simulink model "DoubleTank_PID"  (Simulink 8.1)
settings: Solver=ode4  StartTime=0.0  StopTime=2000  FixedStep=0.5  RelTol=1e-3
PreLoadFcn:
  | pid6=readfis('pid6.fis')
InitFcn:
  | init
settings Model: Creator=Administrator  LastModifiedBy=Administrator
settings DataIOCC: SignalLoggingSaveFormat=Dataset
settings OptimizationCC: ExpressionDepthLimit=128
settings DebuggingCC: FcnCallInpInsideContextMsg=EnableAllAsError
settings GRTTargetCC: CombineOutputUpdateFcns=on  GRTInterface=off

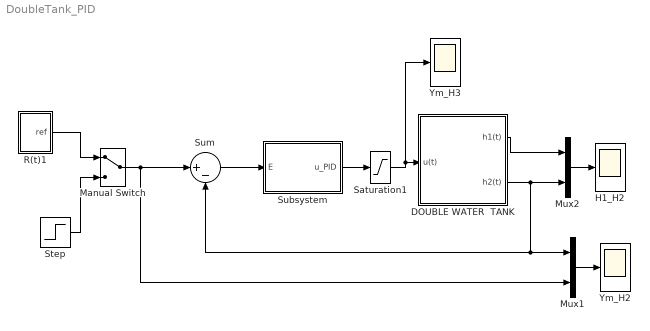
== system DoubleTank_PID ==
  DOUBLE WATER  TANK : Subsystem  mask(Input value){k=6, A_1=15.9043, A_2=15.9043, a1=0.3167, a2=0.1780, g=981}
      mask prompts: k "He so luu luong cua bom k"; A_1 "Tiet dien bon 1"; A_2 "Tiet dien bon 2"; a1 "tiet dien van xa 1"; a2 "tiet dien van xa 2"; g "Gia toc trong truong g"
      mask help: Please input behind values...
  H1_H2 : Scope
      settings: TimeRange=500  YMin=0  YMax=25  SaveName=h1
  Manual Switch : ManualSwitch
  Mux1 : Mux  Inputs=2
  Mux2 : Mux  Inputs=2
  R(t)1 : Subsystem
  Saturation1 : Saturate  UpperLimit=12  LowerLimit=0
  Step : Step  Time=0  After=25  SampleTime=0
  Subsystem : Subsystem  mask{Kp=5, Ki=0.5, Kd=0.1}
      mask prompts: Kp "He so Kp"; Ki "He so Ki"; Kd "He so Kd"
  Sum : Sum  Inputs=|+-
  Ym_H2 : Scope
      settings: TimeRange=500  YMin=38  YMax=42  SaveName=h
  Ym_H3 : Scope
      settings: TimeRange=500  YMin=0  YMax=25  SaveName=h2
  wires:
  Mux2/1 -> H1_H2/1
  R(t)1/1(ref) -> Manual Switch/1
  Step/1 -> Manual Switch/2
  Manual Switch/1 -> Sum/1, Mux1/2
  Subsystem/1(u_PID) -> Saturation1/1
  DOUBLE WATER  TANK/2(h2(t)) -> Mux2/2, Sum/2, Mux1/1
  DOUBLE WATER  TANK/1(h1(t)) -> Mux2/1
  Mux1/1 -> Ym_H2/1
  Saturation1/1 -> Ym_H3/1, DOUBLE WATER  TANK/1(u(t))
  Sum/1 -> Subsystem/1(E)

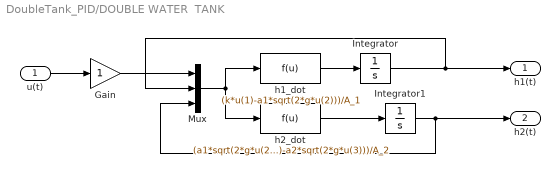
== system DoubleTank_PID/DOUBLE WATER  TANK ==
  u(t) : Inport
  Gain : Gain  SaturateOnIntegerOverflow=on  OutDataTypeStr=Inherit: Same as input  ParamDataTypeStr=Inherit: Same as input
  Integrator : Integrator  LimitOutput=on  UpperSaturationLimit=100  LowerSaturationLimit=0
  Integrator1 : Integrator  LimitOutput=on  UpperSaturationLimit=100  LowerSaturationLimit=0
  Mux : Mux  Inputs=3
  h1_dot : Fcn  Expr=(k*u(1)-a1*sqrt(2*g*u(2)))/A_1
  h2_dot : Fcn  Expr=(a1*sqrt(2*g*u(2))-a2*sqrt(2*g*u(3)))/A_2
  h1(t) : Outport
  h2(t) : Outport  Port=2
  wires:
  h2_dot/1 -> Integrator1/1
  Integrator/1 -> Mux/2, h1(t)/1
  h1_dot/1 -> Integrator/1
  Mux/1 -> h2_dot/1, h1_dot/1
  Integrator1/1 -> Mux/3, h2(t)/1
  u(t)/1 -> Gain/1
  Gain/1 -> Mux/1

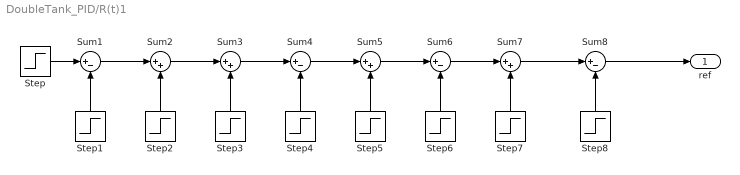
== system DoubleTank_PID/R(t)1 ==
  Step : Step  Time=0  After=15  SampleTime=0
  Step1 : Step  Time=250  After=5  SampleTime=0
  Step2 : Step  Time=500  After=5  SampleTime=0
  Step3 : Step  Time=750  After=15  SampleTime=0
  Step4 : Step  Time=1000  After=10  SampleTime=0
  Step5 : Step  Time=1250  After=15  SampleTime=0
  Step6 : Step  Time=1500  After=5  SampleTime=0
  Step7 : Step  Time=1750  After=15  SampleTime=0
  Step8 : Step  Time=2000  After=5  SampleTime=0
  Sum{1,4,6,8} (4 alike) : Sum  Inputs=|+-  SaturateOnIntegerOverflow=on
  Sum{2..3,5,7} (4 alike) : Sum  Inputs=|++  SaturateOnIntegerOverflow=on
  ref : Outport
  wires:
  Sum5/1 -> Sum6/1
  Step7/1 -> Sum7/2
  Sum6/1 -> Sum7/1
  Step6/1 -> Sum6/2
  Sum3/1 -> Sum4/1
  Step5/1 -> Sum5/2
  Sum4/1 -> Sum5/1
  Step4/1 -> Sum4/2
  Step3/1 -> Sum3/2
  Sum2/1 -> Sum3/1
  Step2/1 -> Sum2/2
  Sum1/1 -> Sum2/1
  Step1/1 -> Sum1/2
  Step/1 -> Sum1/1
  Step8/1 -> Sum8/2
  Sum8/1 -> ref/1
  Sum7/1 -> Sum8/1

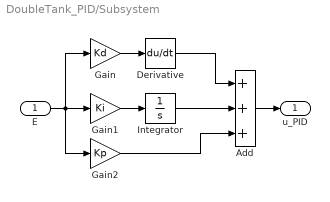
== system DoubleTank_PID/Subsystem ==
  E : Inport
  Add : Sum  Inputs=+++
  Derivative : Derivative
  Gain : Gain  Gain=Kd
  Gain1 : Gain  Gain=Ki
  Gain2 : Gain  Gain=Kp
  Integrator : Integrator
  u_PID : Outport
  wires:
  Derivative/1 -> Add/1
  Integrator/1 -> Add/2
  Gain2/1 -> Add/3
  Gain/1 -> Derivative/1
  Gain1/1 -> Integrator/1
  Add/1 -> u_PID/1
  E/1 -> Gain2/1, Gain/1, Gain1/1
